simulink model "Level2"  (R2021a)
settings: Solver=VariableStepAuto  StartTime=0.0  StopTime=10.0  RelTol=1e-3
values from neighbouring files (symbols this model uses):
  b_PID_hoist = -MEh * nh * wh    (= -542577.777778)    [Data.m]
  b_PID_trolley = MEtd*ntd*wtd    (= 540180)    [Data.m]
  bEh = 2*(bhd + bhm*ih^2)/rhd^2    (= 31004.4444444)    [Data.m]
  bEtd = (btd + btm*it^2)/rtd^2    (= 21607.2)    [Data.m]
  ih = 22    [Data.m]
  it = 30    [Data.m]
  Ksa_PID_hoist = -MEh * nh * wh^2    (= -1807802.81417)    [Data.m]
  Ksa_PID_trolley = MEtd*ntd*wtd^2    (= 3890592.432)    [Data.m]
  Ksia_PID_hoist = -MEh * nh * wh^3    (= -6023377.93542)    [Data.m]
  Ksia_PID_trolley = MEtd*ntd*wtd^3    (= 28021602.9322)    [Data.m]
  rhd = 0.75    [Data.m]
  rtd = 0.5    [Data.m]
settings Model: Creator=jpss8  LastModifiedBy=jpss8

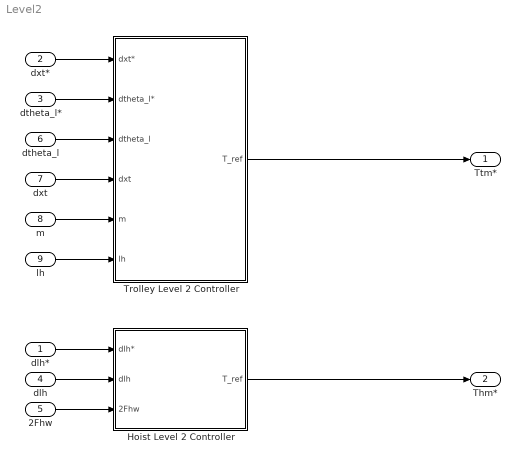
== system Level2 ==
  dlh* : Inport
  dxt* : Inport  Port=2
  dtheta_l* : Inport  Port=3
  dlh : Inport  Port=4
  2Fhw : Inport  Port=5
  dtheta_l : Inport  Port=6
  dxt : Inport  Port=7
  m : Inport  Port=8
  lh : Inport  Port=9
  Hoist Level 2 Controller : Subsystem
  Trolley Level 2 Controller : Subsystem
  Ttm* : Outport
  Thm* : Outport  Port=2
  wires:
  dtheta_l*/1 -> Trolley Level 2 Controller/2(dtheta_l*)
  2Fhw/1 -> Hoist Level 2 Controller/3(2Fhw)
  dlh/1 -> Hoist Level 2 Controller/2(dlh)
  lh/1 -> Trolley Level 2 Controller/6(lh)
  m/1 -> Trolley Level 2 Controller/5(m)
  dxt/1 -> Trolley Level 2 Controller/4(dxt)
  dtheta_l/1 -> Trolley Level 2 Controller/3(dtheta_l)
  Trolley Level 2 Controller/1(T_ref) -> Ttm*/1
  Hoist Level 2 Controller/1(T_ref) -> Thm*/1
  dlh*/1 -> Hoist Level 2 Controller/1(dlh*)
  dxt*/1 -> Trolley Level 2 Controller/1(dxt*)

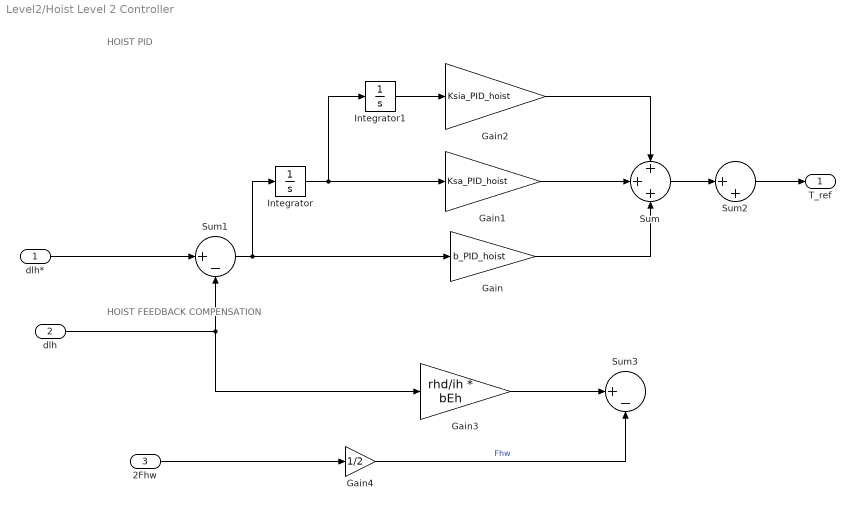
== system Level2/Hoist Level 2 Controller ==
  note: HOIST FEEDBACK COMPENSATION
  note: HOIST PID
  dlh* : Inport
  dlh : Inport  Port=2
  2Fhw : Inport  Port=3
  Gain : Gain  Gain=b_PID_hoist
  Gain1 : Gain  Gain=Ksa_PID_hoist
  Gain2 : Gain  Gain=Ksia_PID_hoist
  Gain3 : Gain  Gain=rhd/ih * bEh
  Gain4 : Gain  Gain=1/2
  Integrator : Integrator
  Integrator1 : Integrator
  Sum : Sum  Inputs=+++
  Sum1 : Sum  Inputs=|+-
  Sum2 : Sum  Inputs=|++
  Sum3 : Sum  Inputs=|+-
  T_ref : Outport
  wires:
  Integrator/1 -> Integrator1/1, Gain1/1
  Integrator1/1 -> Gain2/1
  Gain1/1 -> Sum/2
  Gain2/1 -> Sum/1
  Gain/1 -> Sum/3
  Sum1/1 -> Gain/1, Integrator/1
  Sum2/1 -> T_ref/1
  Sum/1 -> Sum2/1
  Gain3/1 -> Sum3/1
  2Fhw/1 -> Gain4/1
  Gain4/1 -> Sum3/2  "Fhw"
  dlh/1 -> Gain3/1, Sum1/2
  dlh*/1 -> Sum1/1

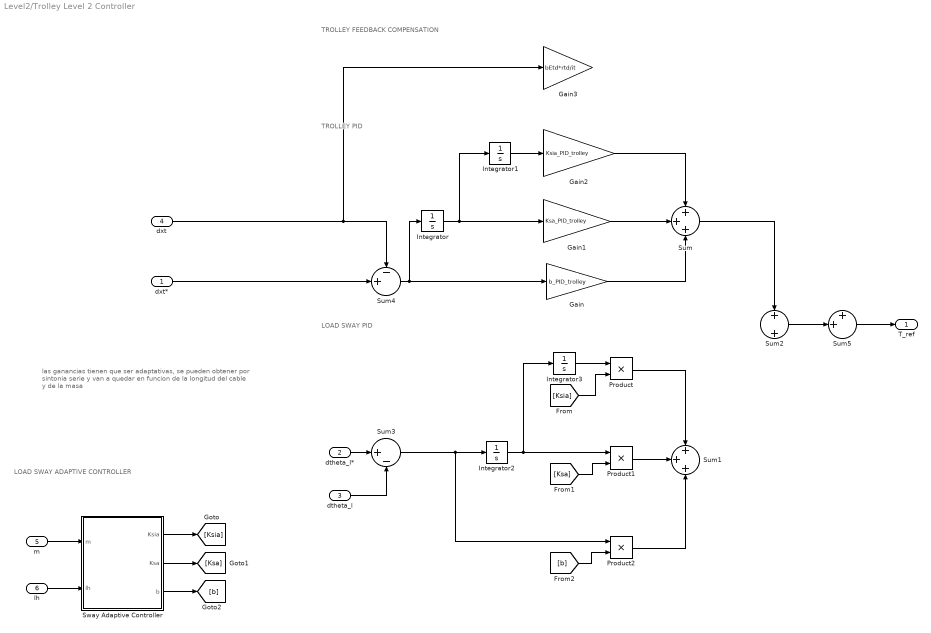
== system Level2/Trolley Level 2 Controller ==
  note: LOAD SWAY ADAPTIVE CONTROLLER
  note: LOAD SWAY PID
  note: TROLLEY FEEDBACK COMPENSATION
  note: TROLLEY PID
  note: las ganancias tienen que ser adaptativas, se pueden obtener por sintonia serie y van a quedar en funcion de la longitud del cable y de la masa
  dxt* : Inport
  dtheta_l* : Inport  Port=2
  dtheta_l : Inport  Port=3
  dxt : Inport  Port=4
  m : Inport  Port=5
  lh : Inport  Port=6
  Gain : Gain  Gain=b_PID_trolley
  Gain1 : Gain  Gain=Ksa_PID_trolley
  Gain2 : Gain  Gain=Ksia_PID_trolley
  Gain3 : Gain  Gain=bEtd*rtd/it
  Integrator{,1..3} (4 alike) : Integrator
  Product : Product
  Product1 : Product
  Product2 : Product
  Sum : Sum  Inputs=+++
  Sum1 : Sum  Inputs=+++
  Sum2 : Sum  Inputs=+|+
  Sum3 : Sum  Inputs=|+-
  Sum4 : Sum  Inputs=-+|
  Sum5 : Sum  Inputs=++|
  Sway Adaptive Controller : Subsystem
  T_ref : Outport
  wires:
  Sum/1 -> Sum2/1
  Gain/1 -> Sum/3
  Gain2/1 -> Sum/1
  Gain1/1 -> Sum/2
  Integrator1/1 -> Gain2/1
  Integrator/1 -> Integrator1/1, Gain1/1
  dtheta_l*/1 -> Sum3/1
  Product2/1 -> Sum1/3
  Integrator2/1 -> Integrator3/1, Product1/1
  Integrator3/1 -> Product/1
  Product1/1 -> Sum1/2
  Product/1 -> Sum1/1
  Sway Adaptive Controller/1(Ksia) -> [Ksia]
  Sway Adaptive Controller/2(Ksa) -> [Ksa]
  Sway Adaptive Controller/3(b) -> [b]
  [Ksia] -> Product/2
  [Ksa] -> Product1/2
  [b] -> Product2/2
  Sum3/1 -> Product2/1, Integrator2/1
  dtheta_l/1 -> Sum3/2
  Sum4/1 -> Integrator/1, Gain/1
  lh/1 -> Sway Adaptive Controller/2(lh)
  m/1 -> Sway Adaptive Controller/1(m)
  Sum5/1 -> T_ref/1
  Sum2/1 -> Sum5/2
  dxt/1 -> Gain3/1, Sum4/1
  dxt*/1 -> Sum4/2

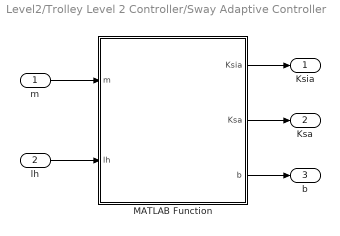
== system Level2/Trolley Level 2 Controller/Sway Adaptive Controller ==
  m : Inport
  lh : Inport  Port=2
  MATLAB Function : MATLAB Function  TreatAsAtomicUnit=on
  Ksia : Outport
  Ksa : Outport  Port=2
  b : Outport  Port=3
  wires:
  m/1 -> MATLAB Function/1(m)
  lh/1 -> MATLAB Function/2(lh)
  MATLAB Function/1(Ksia) -> Ksia/1
  MATLAB Function/2(Ksa) -> Ksa/1
  MATLAB Function/3(b) -> b/1

== matlab function Level2/Trolley Level 2 Controller/Sway Adaptive Controller/MATLAB Function ==
  data: m input; Ksia output; lh input; Ksa output; b output
function [Ksia, Ksa, b] = get_sway_adaptive_gains(m, lh)

Ksia = 1;
Ksa = 1;
b = 1;

end
